simulink model "simplificado"  (R2023a)
settings: Solver=VariableStepAuto  StartTime=0.0  StopTime=400  RelTol=1e-3
values from neighbouring files (symbols this model uses):
  A1 = 0.0154    [expert_pid_script.m]    (also in optimizer.m; parametros.m; variables.mat)
  A2 = 5e-5    (= 5e-05)    [expert_pid_script.m]    (also in optimizer.m; parametros.m; variables.mat)
  az = 1    [expert_pid_script.m]    (also in optimizer.m; parametros.m = 0.5; variables.mat = 0.5)
  g = 9.8    [expert_pid_script.m]    (also in optimizer.m; parametros.m; variables.mat)
  H_star = H_max/2    (= 0.31)    [expert_pid_script.m]    (also in optimizer.m; parametros.m; variables.mat)
  ro = 1000    [expert_pid_script.m]    (also in optimizer.m; parametros.m; variables.mat)
  st = 0.001    [parametros.m]    (also in variables.mat)
undefined symbols (not defined in the file or in its folder): DiscIntNeverNeededParam
settings Model: Creator=empg0  LastModifiedBy=empg0
settings DebuggingCC: AlgebraicLoopMsg=none

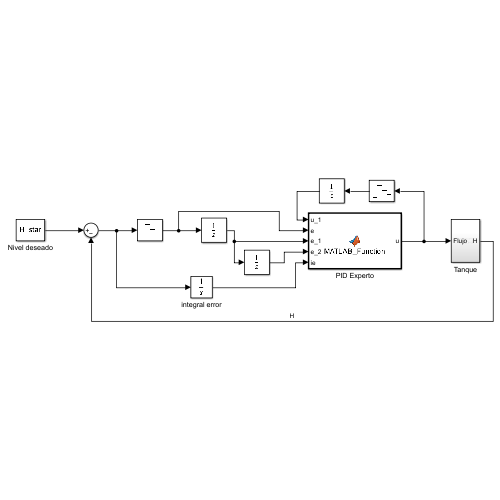
[thumbnail: Simulink's stored preview of the top-level diagram]
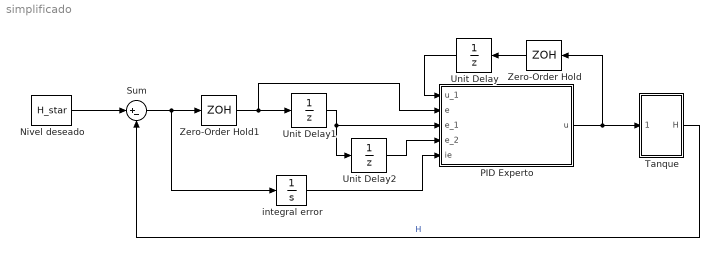
== system simplificado ==
  Nivel deseado : Constant  Value=H_star
  PID Experto : MATLAB Function  TreatAsAtomicUnit=on
  Sum : Sum  Inputs=|+-
  Tanque : Subsystem
  Unit Delay : UnitDelay  SampleTime=st  HasFrameUpgradeWarning=on
  Unit Delay1 : UnitDelay  SampleTime=st  HasFrameUpgradeWarning=on
  Unit Delay2 : UnitDelay  SampleTime=st  HasFrameUpgradeWarning=on
  Zero-Order Hold : ZeroOrderHold  SampleTime=st
  Zero-Order Hold1 : ZeroOrderHold  SampleTime=st
  integral error : Integrator
  wires:
  Tanque/1(H) -> Sum/2  "H"
  Nivel deseado/1 -> Sum/1
  Sum/1 -> Zero-Order Hold1/1, integral error/1
  Zero-Order Hold1/1 -> Unit Delay1/1, PID Experto/2(e)
  Unit Delay2/1 -> PID Experto/4(e_2)
  Unit Delay1/1 -> Unit Delay2/1, PID Experto/3(e_1)
  integral error/1 -> PID Experto/5(ie)
  PID Experto/1(u) -> Tanque/1(Flujo), Zero-Order Hold/1
  Zero-Order Hold/1 -> Unit Delay/1
  Unit Delay/1 -> PID Experto/1(u_1)

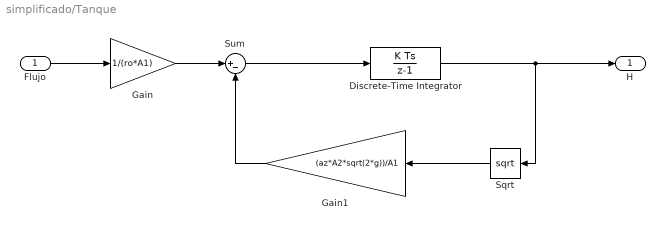
== system simplificado/Tanque ==
  Flujo : Inport
  Discrete-Time Integrator : DiscreteIntegrator  SampleTime=st  LimitOutput=on  UpperSaturationLimit=0.62  LowerSaturationLimit=0  ICPrevOutput=DiscIntNeverNeededParam  ICPrevScaledInput=DiscIntNeverNeededParam
  Gain : Gain  Gain=1/(ro*A1)
  Gain1 : Gain  Gain=(az*A2*sqrt(2*g))/A1
  Sqrt : Sqrt
  Sum : Sum  Inputs=|+-
  H : Outport
  wires:
  Gain/1 -> Sum/1
  Sqrt/1 -> Gain1/1
  Gain1/1 -> Sum/2
  Flujo/1 -> Gain/1
  Sum/1 -> Discrete-Time Integrator/1
  Discrete-Time Integrator/1 -> H/1, Sqrt/1

== matlab function simplificado/PID Experto ==
  data: u_1 input; e input; u output; e_1 input; e_2 input; ie input
function u = MATLAB_Function(u_1, e, e_1, e_2, ie)
    
    %st = load("sampling_time.mat");
    % Constantes
    H_max = 0.62;
    M1 = H_max/2;
    M2 = H_max/4;
    epsilon = 0.001; % cambié de 0.01 a 0.005
    st = 0.001; % 0.1 -> 0.001

    Qmax = 0.1; % flujo máximo
    Qmin = 0; % flujo mínimo
    
    k1 = 4.9321;
    k2 = 0.033265;
    kp = 1.06160;
    ki = 0.05; %0.03014;
    kd = -2.20023;

    de = e - e_1;
    de_1 = e_1 - e_2;
    if abs(e) > M1 % regla 1
        r = 1;
        if e > 0
            u = Qmax;
        else
            u = Qmin;
        end
    elseif abs(e) <= epsilon % regla 5
        r = 5;
        u = u_1 + kp*(e - e_1) + ki*ie;
    elseif e*de < 0 && de*de_1 < 0 % regla 4
        r = 4;
        if abs(e) >= M2
            u = u_1 + k1*kp*e;
        else
            u = u_1 + k2*kp*e;
        end
    elseif (e*de < 0 && de*de_1 > 0) || e == 0 % regla 3
        r = 3;
        u = u_1;
    elseif e*de > 0 || de == 0 % regla 2
        % funcionaba mejor cuando la regla 2 era pid normal
        r = 2;
        if abs(e) >= M2
            %control fuerte
            u = u_1 + k1*kp*(e - e_1) + k1*ki*e + k1*kd*(e - 2*e_1 + e_2);
        else
            %control débil
            u = u_1 + kp*(e - e_1) + ki*e + kd*(e - 2*e_1 + e_2);
        end
    else
        r = 0;
        u = kp*e + (kd*de)/st + ki*ie;
    end
    if u > 0.1
        u = 0.1;
    end
    if u < 0
        u = 0;
    end
